simulink model "NoThermalControl"  (R2024b)
settings: configuration reference "VehicleFixed100ms" (kept outside this file)
settings Model: DataDictionary=VirtualVehicleTemplate.sldd  ModifiedByFormat=The MathWorks, Inc.  Creator=The MathWorks, Inc.  LastModifiedBy=The MathWorks, Inc.
settings ConfigSetRef: SourceName=VehicleFixed100ms

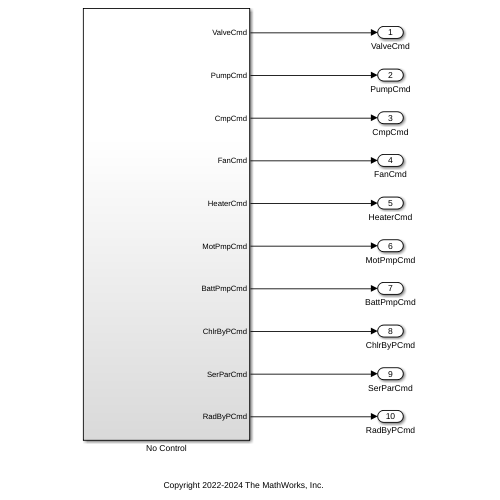
[thumbnail: Simulink's stored preview of the top-level diagram]
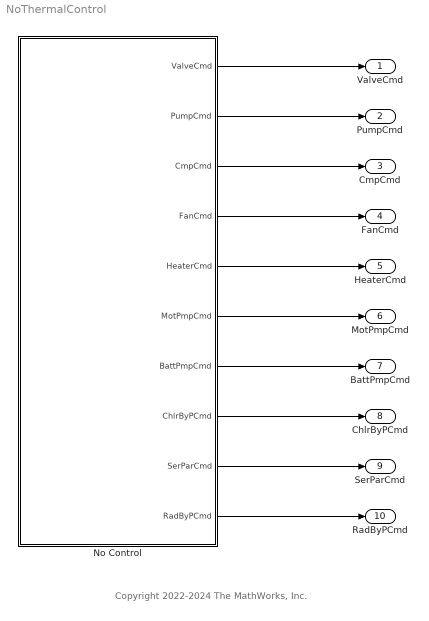
== system NoThermalControl ==
  note: Copyright 2022-2024 The MathWorks, Inc.
  No Control : Subsystem  VariantControl=No Control
  ValveCmd : Outport
  PumpCmd : Outport  Port=2
  CmpCmd : Outport  Port=3
  FanCmd : Outport  Port=4
  HeaterCmd : Outport  Port=5
  MotPmpCmd : Outport  Port=6
  BattPmpCmd : Outport  Port=7
  ChlrByPCmd : Outport  Port=8
  SerParCmd : Outport  Port=9
  RadByPCmd : Outport  Port=10
  wires:
  No Control/1(ValveCmd) -> ValveCmd/1
  No Control/2(PumpCmd) -> PumpCmd/1
  No Control/3(CmpCmd) -> CmpCmd/1
  No Control/4(FanCmd) -> FanCmd/1
  No Control/5(HeaterCmd) -> HeaterCmd/1
  No Control/6(MotPmpCmd) -> MotPmpCmd/1
  No Control/7(BattPmpCmd) -> BattPmpCmd/1
  No Control/8(ChlrByPCmd) -> ChlrByPCmd/1
  No Control/9(SerParCmd) -> SerParCmd/1
  No Control/10(RadByPCmd) -> RadByPCmd/1

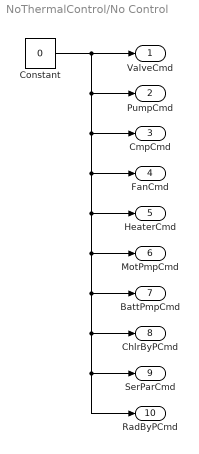
== system NoThermalControl/No Control ==
  Constant : Constant  Value=0  SampleTime=-1
  ValveCmd : Outport
  PumpCmd : Outport  Port=2
  CmpCmd : Outport  Port=3
  FanCmd : Outport  Port=4
  HeaterCmd : Outport  Port=5
  MotPmpCmd : Outport  Port=6
  BattPmpCmd : Outport  Port=7
  ChlrByPCmd : Outport  Port=8
  SerParCmd : Outport  Port=9
  RadByPCmd : Outport  Port=10
  wires:
  Constant/1 -> ValveCmd/1, RadByPCmd/1, SerParCmd/1, ChlrByPCmd/1, BattPmpCmd/1, MotPmpCmd/1, HeaterCmd/1, FanCmd/1, CmpCmd/1, PumpCmd/1
